simulink model "wind_pmsg_vsc_pv"  (R2024a)
settings: Solver=VariableStepAuto  StartTime=0.0  StopTime=5  RelTol=1e-3
undefined symbols (not defined in the file): D1, Delta, Ion, Lithium, Ts_Control
libraries: spsSeriesRLCBranchLib x13, spsDiodeLib x10, slpidlib x7, spsCurrentMeasurementLib x6, spsVoltageMeasurementLib x4, spsIdealSwitchLib x3, spsPWMGeneratorDCDCLib x3, eeStairGenerator x3, spsBreakerLib x2, spsThreePhaseVIMeasurementLib x2, spsabctodq0Lib x2, spsThreePhaseTransformerTwoWindingsLib x2
(part 2 of 2)

== matlab function wind_pmsg_vsc_pv/MPPT/MATLAB Function ==
  settings: updateMethod=DISCRETE
  data: Param input; D output; Enabled input; V input; I input
function D  = PandO(Param, Enabled, V, I)

% MPPT controller based on the Perturb & Observe algorithm.

% D output = Reference for DC link voltage (Vdc_ref) 
%
% Enabled input = 1 to enable the MPPT controller
% V input = PV array terminal voltage (V)
% I input = PV array current (A)
%
% Param input:
Dinit = Param(1);  %Initial value for Vdc_ref
Dmax = Param(2);   %Maximum value for Vdc_ref
Dmin = Param(3);   %Minimum value for Vdc_ref
deltaD = Param(4); %Increment value used to increase/decrease Vdc_ref
%  

persistent Vold Pold Dold;

dataType = 'double';

if isempty(Vold)
    Vold=0;
    Pold=0;
    Dold=Dinit;
end
P= V*I;
dV= V - Vold;
dP= P - Pold;

if dP ~= 0 & Enabled ~=0
    if dP < 0
        if dV < 0
            D = Dold + deltaD;
        else
            D = Dold - deltaD;
        end
    else
        if dV < 0
            D = Dold - deltaD;
        else
            D = Dold + deltaD;
        end    
    end
else D=Dold;
end

if D >= Dmax | D<= Dmin
    D=Dold;
end

Dold=D;
Vold=V;
Pold=P;

== matlab function wind_pmsg_vsc_pv/Subsystem3/MATLAB Function2 ==
  data: ibat1 input; y output; ibat2 input; t input
function y = fcn(ibat1, ibat2,t)
if t<=3
    y= ibat1;
else 
    y= ibat2;
end
